simulink model "mcb_param_est_sensorless_nucleo_g474re_ihm07m1"  (R2024a)
settings: Solver=FixedStepDiscrete  StartTime=0.0  StopTime=Inf  FixedStep=Ts  RelTol=1e-3  EnableMultiTasking=on
model workspace (MAT data in the model file):
  encoderResolution = 2000
  hallOffset = '0.5'
  indexOffset = 850
  polePairs = '4'
values from neighbouring files (symbols this model uses):
  PWM_Counter_Period = round(CPU_frequency/PWM_frequency/2)    [mcb_stm32_param_est_InitFunc.m]
  Ts = 1/PWM_frequency    (= 5e-05)    [mcb_stm32_param_est_InitFunc.m]
undefined symbols (not defined in the file or in its folder): DiscIntNeverNeededParam, inverter, motorParam, NumBits1, NumBits2, Slope1, Slope2
libraries: mcbcontrolslib x24, simulink x15, stm32f4xxblockslib x5, stm32g4xxblockslib x4, slpidlib x2, stm32blockslib x2, svdutilitieslib x1
(part 3 of 3)

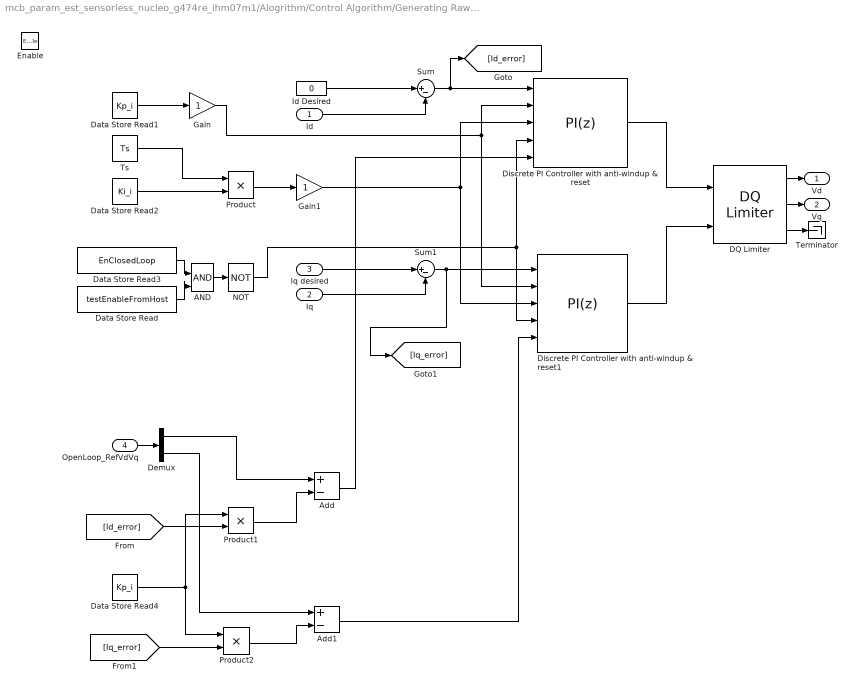
== system mcb_param_est_sensorless_nucleo_g474re_ihm07m1/Alogrithm/Control Algorithm/Generating Raw Space Vectors/OpenLoop_CloseLoop/Control ==
  Id : Inport
  Iq : Inport  Port=2
  Iq desired : Inport  Port=3
  OpenLoop_RefVdVq : Inport  Port=4
  Enable : EnablePort
  AND : Logic  IconShape=distinctive  AllPortsSameDT=off  OutDataTypeStr=boolean
  Add : Sum  Inputs=+-  OutDataTypeStr=single  AccumDataTypeStr=single
  Add1 : Sum  Inputs=+-  OutDataTypeStr=single  AccumDataTypeStr=single
  DQ Limiter : mcbcontrolslib/DQ Limiter  satMethodInputType=Specify via dialog  satMethodSelected=D-Q equivalence  satLimitInputType=Specify via dialog  Vmax=0.95
  Data Store Read : DataStoreRead  DataStoreName=testEnableFromHost  IndexOptions=Index vector (dialog)  Indices=1  OutputSizes=1
  Data Store Read1 : DataStoreRead  DataStoreName=Kp_i  IndexOptions=Index vector (dialog)  Indices=1  OutputSizes=1
  Data Store Read2 : DataStoreRead  DataStoreName=Ki_i  IndexOptions=Index vector (dialog)  Indices=1  OutputSizes=1
  Data Store Read4 : DataStoreRead  DataStoreName=Kp_i  IndexOptions=Index vector (dialog)  Indices=1  OutputSizes=1
  Data Store Read3 : DataStoreRead  DataStoreName=EnClosedLoop  IndexOptions=Index vector (dialog)  Indices=1  OutputSizes=1
  Demux : Demux  Outputs=2
  Discrete PI Controller with anti-windup & reset : slpidlib/PID Controller  Controller=PI  Form=Parallel  TimeDomain=Discrete-time  UseExternalTs=off  SampleTime=-1  IntegratorMethod=Forward Euler  FilterMethod=Forward Euler  ControllerParametersSource=external  P=1  I=1  UseKiTs=on  D=0  UseExternalDerivativeSource=off  N=100  UseFilter=on  TunerSelectOption=Transfer Function Based (PID Tuner App)  InitialConditionSource=external  InitialConditionForIntegrator=0  InitialConditionForFilter=0  DifferentiatorICPrevScaledInput=0  ExternalReset=level  TrackingMode=off  Kt=1  LimitOutput=on  SatLimitsSource=internal  UpperSaturationLimit=1  LowerSaturationLimit=-1  LinearizeAsGain=on  AntiWindupMode=clamping  Kb=1  LimitIntegrator=off  UpperIntegratorSaturationLimit=inf  LowerIntegratorSaturationLimit=-inf  RndMeth=Simplest  POutMin=[]  POutMax=[]  IOutMin=[]  IOutMax=[]  DOutMin=[]  DOutMax=[]  NOutMin=[]  NOutMax=[]  SumOutMin=[]  SumOutMax=[]  SaturationOutDataTypeStr=Inherit: Inherit via back propagation  SaturationOutMin=[]  SaturationOutMax=[]  PParamMin=[]  PParamMax=[]  IParamMin=[]  IParamMax=[]  DParamMin=[]  DParamMax=[]  NParamMin=[]  NParamMax=[]  KbParamMin=[]  KbParamMax=[]  KtParamMin=[]  KtParamMax=[]  KbOutMin=[]  KbOutMax=[]  KtOutMin=[]  KtOutMax=[]  IntegratorOutMin=[]  IntegratorOutMax=[]  FilterOutMin=[]  FilterOutMax=[]  SumI1OutMin=[]  SumI1OutMax=[]  SumI2OutMin=[]  SumI2OutMax=[]  SumI3OutMin=[]  SumI3OutMax=[]  SumI4OutMin=[]  SumI4OutMax=[]  SumDOutMin=[]  SumDOutMax=[]  DifferentiatorOutMin=[]  DifferentiatorOutMax=[]  FilterDiffOutCoefMin=[]  FilterDiffOutCoefMax=[]  ReciprocalOutMin=[]  ReciprocalOutMax=[]  SumDenOutMin=[]  SumDenOutMax=[]  SumNumOutMin=[]  SumNumOutMax=[]  DivideOutMin=[]  DivideOutMax=[]  UdiffTsProdOutMin=[]  UdiffTsProdOutMax=[]  NTsProdOutMin=[]  NTsProdOutMax=[]  UintegralTsProdOutMin=[]  UintegralTsProdOutMax=[]  UngainTsProdOutMin=[]  UngainTsProdOutMax=[]  ClampingZeroOutDataTypeStr=Inherit: Inherit via back propagation  ClampingZeroOutMin=[]  ClampingZeroOutMax=[]  FilterDenConstantOutDataTypeStr=Inherit: Inherit via back propagation  FilterDenConstantOutMin=[]  FilterDenConstantOutMax=[]  PCopyOutDataTypeStr=Inherit: Inherit via back propagation  PCopyOutMin=[]  PCopyOutMax=[]  NCopyOutDataTypeStr=Inherit: Inherit via back propagation  NCopyOutMin=[]  NCopyOutMax=[]  IntegratorContinuousStateAttributes=''  IntegratorStateMustResolveToSignalObject=off  IntegratorRTWStateStorageClass=Auto  FilterContinuousStateAttributes=''  FilterStateMustResolveToSignalObject=off  FilterRTWStateStorageClass=Auto  ParallelPVariant=ExternalParameters  IdealPVariant=Disabled  IVariant=ExternalParameters  DVariant=Disabled  IntegratorVariant=Discrete  SatVariant=Enabled  AWVariant=DiscClampingParallel  PCopyVariant=Disabled  TRVariant=Disabled  FdbkBlocksVariant=Forward  IdealPFdbkVariant=Disabled  SatFdbkVariant=Disabled  DerivativeFilterVariant=Disabled  NVariant=Disabled  NCopyVariant=Disabled_SignalSpec  FilterICVariant=Disabled  IntegratorICVariant=ExternalICs  ExternalResetVariant=ExternalReset  TRSumVariant=Passthrough  SumFdbkVariant=Disabled  SumVariant=Sum_PI  TsampFilterVariant=InternalTs  TsampNgainVariant=Passthrough  TsampIntegralVariant=Disabled_SignalSpec  ExternalSaturationOutDataTypeStr=Inherit: Same as second input  DerivativeSourceVariant=Disabled
  Discrete PI Controller with anti-windup & reset1 : slpidlib/PID Controller  Controller=PI  Form=Parallel  TimeDomain=Discrete-time  UseExternalTs=off  SampleTime=-1  IntegratorMethod=Forward Euler  FilterMethod=Forward Euler  ControllerParametersSource=external  P=1  I=1  UseKiTs=on  D=0  UseExternalDerivativeSource=off  N=100  UseFilter=on  TunerSelectOption=Transfer Function Based (PID Tuner App)  InitialConditionSource=external  InitialConditionForIntegrator=0  InitialConditionForFilter=0  DifferentiatorICPrevScaledInput=0  ExternalReset=level  TrackingMode=off  Kt=1  LimitOutput=on  SatLimitsSource=internal  UpperSaturationLimit=1  LowerSaturationLimit=-1  LinearizeAsGain=on  AntiWindupMode=clamping  Kb=1  LimitIntegrator=off  UpperIntegratorSaturationLimit=inf  LowerIntegratorSaturationLimit=-inf  RndMeth=Simplest  POutMin=[]  POutMax=[]  IOutMin=[]  IOutMax=[]  DOutMin=[]  DOutMax=[]  NOutMin=[]  NOutMax=[]  SumOutMin=[]  SumOutMax=[]  SaturationOutDataTypeStr=Inherit: Inherit via back propagation  SaturationOutMin=[]  SaturationOutMax=[]  PParamMin=[]  PParamMax=[]  IParamMin=[]  IParamMax=[]  DParamMin=[]  DParamMax=[]  NParamMin=[]  NParamMax=[]  KbParamMin=[]  KbParamMax=[]  KtParamMin=[]  KtParamMax=[]  KbOutMin=[]  KbOutMax=[]  KtOutMin=[]  KtOutMax=[]  IntegratorOutMin=[]  IntegratorOutMax=[]  FilterOutMin=[]  FilterOutMax=[]  SumI1OutMin=[]  SumI1OutMax=[]  SumI2OutMin=[]  SumI2OutMax=[]  SumI3OutMin=[]  SumI3OutMax=[]  SumI4OutMin=[]  SumI4OutMax=[]  SumDOutMin=[]  SumDOutMax=[]  DifferentiatorOutMin=[]  DifferentiatorOutMax=[]  FilterDiffOutCoefMin=[]  FilterDiffOutCoefMax=[]  ReciprocalOutMin=[]  ReciprocalOutMax=[]  SumDenOutMin=[]  SumDenOutMax=[]  SumNumOutMin=[]  SumNumOutMax=[]  DivideOutMin=[]  DivideOutMax=[]  UdiffTsProdOutMin=[]  UdiffTsProdOutMax=[]  NTsProdOutMin=[]  NTsProdOutMax=[]  UintegralTsProdOutMin=[]  UintegralTsProdOutMax=[]  UngainTsProdOutMin=[]  UngainTsProdOutMax=[]  ClampingZeroOutDataTypeStr=Inherit: Inherit via back propagation  ClampingZeroOutMin=[]  ClampingZeroOutMax=[]  FilterDenConstantOutDataTypeStr=Inherit: Inherit via back propagation  FilterDenConstantOutMin=[]  FilterDenConstantOutMax=[]  PCopyOutDataTypeStr=Inherit: Inherit via back propagation  PCopyOutMin=[]  PCopyOutMax=[]  NCopyOutDataTypeStr=Inherit: Inherit via back propagation  NCopyOutMin=[]  NCopyOutMax=[]  IntegratorContinuousStateAttributes=''  IntegratorStateMustResolveToSignalObject=off  IntegratorRTWStateStorageClass=Auto  FilterContinuousStateAttributes=''  FilterStateMustResolveToSignalObject=off  FilterRTWStateStorageClass=Auto  ParallelPVariant=ExternalParameters  IdealPVariant=Disabled  IVariant=ExternalParameters  DVariant=Disabled  IntegratorVariant=Discrete  SatVariant=Enabled  AWVariant=DiscClampingParallel  PCopyVariant=Disabled  TRVariant=Disabled  FdbkBlocksVariant=Forward  IdealPFdbkVariant=Disabled  SatFdbkVariant=Disabled  DerivativeFilterVariant=Disabled  NVariant=Disabled  NCopyVariant=Disabled_SignalSpec  FilterICVariant=Disabled  IntegratorICVariant=ExternalICs  ExternalResetVariant=ExternalReset  TRSumVariant=Passthrough  SumFdbkVariant=Disabled  SumVariant=Sum_PI  TsampFilterVariant=InternalTs  TsampNgainVariant=Passthrough  TsampIntegralVariant=Disabled_SignalSpec  ExternalSaturationOutDataTypeStr=Inherit: Same as second input  DerivativeSourceVariant=Disabled
  Gain : Gain  OutDataTypeStr=Inherit: Same as input  ParamDataTypeStr=Inherit: Same as input
  Gain1 : Gain  OutDataTypeStr=Inherit: Same as input  ParamDataTypeStr=Inherit: Same as input
  Id Desired : Constant  Value=0  OutDataTypeStr=single
  NOT : Logic  Operator=NOT  AllPortsSameDT=off  OutDataTypeStr=boolean
  Product : Product  OutDataTypeStr=Inherit: Same as first input
  Product1 : Product  OutDataTypeStr=single
  Product2 : Product  OutDataTypeStr=single
  Sum : Sum  Inputs=|+-
  Sum1 : Sum  Inputs=|+-
  Terminator : Terminator
  Ts : Constant  Value=Ts  OutDataTypeStr=single  SampleTime=-1
  Vd : Outport  VectorParamsAs1DForOutWhenUnconnected=off
  Vq : Outport  Port=2  VectorParamsAs1DForOutWhenUnconnected=off
  wires:
  Id/1 -> Sum/2
  Iq/1 -> Sum1/2
  Iq desired/1 -> Sum1/1
  Id Desired/1 -> Sum/1
  Sum1/1 -> [Iq_error], Discrete PI Controller with anti-windup & reset1/1
  Sum/1 -> [Id_error], Discrete PI Controller with anti-windup & reset/1
  Product/1 -> Gain1/1
  Data Store Read3/1 -> AND/1
  NOT/1 -> Discrete PI Controller with anti-windup & reset/4, Discrete PI Controller with anti-windup & reset1/4
  Data Store Read1/1 -> Gain/1
  Ts/1 -> Product/1
  Data Store Read2/1 -> Product/2
  Discrete PI Controller with anti-windup & reset/1 -> DQ Limiter/1
  Data Store Read/1 -> AND/2
  AND/1 -> NOT/1
  DQ Limiter/1 -> Vd/1
  DQ Limiter/2 -> Vq/1
  DQ Limiter/3 -> Terminator/1
  Discrete PI Controller with anti-windup & reset1/1 -> DQ Limiter/2
  Gain/1 -> Discrete PI Controller with anti-windup & reset/2, Discrete PI Controller with anti-windup & reset1/2
  Gain1/1 -> Discrete PI Controller with anti-windup & reset/3, Discrete PI Controller with anti-windup & reset1/3
  OpenLoop_RefVdVq/1 -> Demux/1
  Demux/2 -> Add1/1
  Demux/1 -> Add/1
  Data Store Read4/1 -> Product1/1, Product2/1
  Product1/1 -> Add/2
  Add/1 -> Discrete PI Controller with anti-windup & reset/5
  Product2/1 -> Add1/2
  Add1/1 -> Discrete PI Controller with anti-windup & reset1/5
  [Id_error] -> Product1/2
  [Iq_error] -> Product2/2

== system mcb_param_est_sensorless_nucleo_g474re_ihm07m1/Alogrithm/Control Algorithm/Generating Raw Space Vectors/OpenLoop_CloseLoop/OpenLoop ==
  TestNum : Inport
  Freq : Inport  Port=2
  RefSignal : Inport  Port=3
  RefSignal_1 : Inport  Port=4
  Enable : EnablePort
  ADC_Calibration : Subsystem
  BiasedSineWaveLdMeas : Subsystem
  Demux : Demux  Outputs=2
  Index Vector : MultiPortSwitch  DataPortOrder=Zero-based contiguous  Inputs=4  zeroidx=on  SaturateOnIntegerOverflow=off  InputSameDT=off
  Rs_Measurement : Subsystem
  SineWaveLqMeas : Subsystem
  RefVd : Outport  VectorParamsAs1DForOutWhenUnconnected=off
  RefVq : Outport  Port=2  VectorParamsAs1DForOutWhenUnconnected=off
  wires:
  Demux/1 -> RefVd/1
  Demux/2 -> RefVq/1
  BiasedSineWaveLdMeas/1(RefVdVq) -> Index Vector/4
  Freq/1 -> SineWaveLqMeas/2(Freq), BiasedSineWaveLdMeas/2(Freq)
  TestNum/1 -> Index Vector/1
  Index Vector/1 -> Demux/1
  Rs_Measurement/1(RefVdVq) -> Index Vector/3  "Rs_Measurement:1"
  ADC_Calibration/1(RefVdVq) -> Index Vector/2  "ADC_Calibration:1"
  RefSignal/1 -> Rs_Measurement/1(Vd_ref), BiasedSineWaveLdMeas/1(Vd_ref), SineWaveLqMeas/1(Vd_ref)
  SineWaveLqMeas/1(RefVdVq) -> Index Vector/5
  RefSignal_1/1 -> SineWaveLqMeas/3(Vdq_amp), BiasedSineWaveLdMeas/3(Vdq_amp)

== system mcb_param_est_sensorless_nucleo_g474re_ihm07m1/Alogrithm/SaveEstParam_Serial Send/Serial Send/AlternateData/Alternate_0_2 ==
  NOT : Logic  Operator=NOT  IconShape=distinctive  AllPortsSameDT=off  OutDataTypeStr=boolean
  Unit Delay : UnitDelay  InitialCondition=1  SampleTime=-1  HasFrameUpgradeWarning=on
  Out1 : Outport
  wires:
  NOT/1 -> Unit Delay/1, Out1/1
  Unit Delay/1 -> NOT/1

== system mcb_param_est_sensorless_nucleo_g474re_ihm07m1/Alogrithm/SaveEstParam_Serial Send/Serial Send/Serial Send/Data ==
  Data : Inport
  Data_width : Inport  Port=2
  Action Port : ActionPort  ActionPortLabel=else
  Mux : Mux  Inputs=2
  Start : Constant  Value=hex2dec('00000000')  OutDataTypeStr=uint32
  Data_out : Outport  VectorParamsAs1DForOutWhenUnconnected=off
  Iteration : Outport  Port=2  VectorParamsAs1DForOutWhenUnconnected=off
  wires:
  Start/1 -> Mux/2
  Mux/1 -> Data_out/1
  Data/1 -> Mux/1
  Data_width/1 -> Iteration/1

== system mcb_param_est_sensorless_nucleo_g474re_ihm07m1/Alogrithm/SaveEstParam_Serial Send/Serial Send/Serial Send/End ==
  Data : Inport
  Data_width : Inport  Port=2
  Action Port : ActionPort  ActionPortLabel=elseif(u1 == 599)
  Bias : Bias  Bias=1  SaturateOnIntegerOverflow=off
  Mux : Mux  Inputs=2
  Start : Constant  Value=hex2dec('45454545')  OutDataTypeStr=uint32
  Data_out : Outport  VectorParamsAs1DForOutWhenUnconnected=off
  Iteration : Outport  Port=2  VectorParamsAs1DForOutWhenUnconnected=off
  wires:
  Mux/1 -> Data_out/1
  Data_width/1 -> Bias/1
  Start/1 -> Mux/2
  Bias/1 -> Iteration/1
  Data/1 -> Mux/1

== system mcb_param_est_sensorless_nucleo_g474re_ihm07m1/Alogrithm/SaveEstParam_Serial Send/Serial Send/Serial Send/Start ==
  Data : Inport
  Data_width : Inport  Port=2
  Action Port : ActionPort  ActionPortLabel=if(u1 == 0)
  Bias : Bias  Bias=1  SaturateOnIntegerOverflow=off
  End : Constant  Value=hex2dec('53535353')  OutDataTypeStr=uint32
  Mux : Mux  Inputs=2
  Data_out : Outport  VectorParamsAs1DForOutWhenUnconnected=off
  Iteration : Outport  Port=2  VectorParamsAs1DForOutWhenUnconnected=off
  wires:
  End/1 -> Mux/1
  Mux/1 -> Data_out/1
  Data_width/1 -> Bias/1
  Bias/1 -> Iteration/1
  Data/1 -> Mux/2

== system mcb_param_est_sensorless_nucleo_g474re_ihm07m1/Alogrithm/SaveEstParam_Serial Send/Serial Send/Serial Send/While Iterator Subsystem ==
  Data : Inport
  Iteration : Inport  Port=2
  Add : Sum  Inputs=+-  OutDataTypeStr=Inherit: Same as first input
  Index Vector : MultiPortSwitch  Inputs=1  SaturateOnIntegerOverflow=off  InputSameDT=off
  UART/USART Write : stm32blockslib/UART//USART Write  Priority=1  UARTModule=LPUART1  LengthOfDataToSend=off  BlockingMode=on  BlockingTimeout=1e-3  OutputStatus=off
  While Iterator : WhileIterator  MaxIters=-1  WhileBlockType=do-while  ShowIterationPort=on  OutputDataType=int16
  wires:
  Iteration/1 -> Add/1
  Add/1 -> While Iterator/1
  Index Vector/1 -> UART/USART Write/1
  Data/1 -> Index Vector/2
  While Iterator/1 -> Index Vector/1, Add/2

== system mcb_param_est_sensorless_nucleo_g474re_ihm07m1/Alogrithm/Control Algorithm/Flux Observer/FluxObvserver/FluxObserverSubsystem/psiAlpha ==
  note: Integrator
  Reset : Inport
  Valpha : Inport  Port=2
  Ialpha : Inport  Port=3
  scaling : Inport  Port=4
  scalingLd : Inport  Port=5
  Data Type Propagation : simulink/Signal Attributes/Data Type Propagation  PropDataType=fixdt(1, 16)  IfRefDouble=double  IfRefSingle=single  IsSigned=IsSigned1 or IsSigned2  NumBitsBase=max([NumBits1 NumBits2])  NumBitsMult=1  NumBitsAdd=0  NumBitsAllowFinal=1:128  PropScalingMode=Obtain via best precision  PropScaling=2^-10  ValuesUsedBestPrec=[4 -4]  SlopeBase=min([Slope1 Slope2])  SlopeMult=1  SlopeAdd=0  BiasBase=Bias1  BiasMult=1  BiasAdd=0
  Delay : Delay  DelayLength=1  ExternalReset=Level
      settings: InputPortMap=u0,r5
  Gain : Gain  Gain=Ts  ParamDataTypeStr=Inherit: Inherit from 'Gain'  OutDataTypeStr=Inherit: Inherit via back propagation
  IIR Filter3 : mcbcontrolslib/IIR Filter  VariantControl=Low Pass Filter  VariantSelect=Low-pass  FilterConstantInputType=Specify via dialog  Filter_constant=0.001*(Ts/(50e-6))  advancedSettings=off  Ts=50e-6  cutOff_freq=1
  Product : Product  RndMeth=Simplest  OutDataTypeStr=Inherit: Same as first input
  Scaling : Subsystem
  Sum : Sum  Inputs=|++
  Sum1 : Sum  Inputs=|+-  RndMeth=Simplest  OutDataTypeStr=Inherit: Same as first input
  Sum3 : Sum  Inputs=|+-  RndMeth=Simplest  OutDataTypeStr=Inherit: Same as first input
  Sum6 : Sum  Inputs=|+-  RndMeth=Simplest  OutDataTypeStr=Inherit: Same as first input
  psiAlpha : Outport
  wires:
  Sum/1 -> Sum1/1, Delay/1
  IIR Filter3/1 -> Sum6/2
  Sum6/1 -> psiAlpha/1
  Valpha/1 -> Scaling/1("Valpha ")
  Ialpha/1 -> Product/1, Scaling/2(Ialpha)
  Scaling/1(ValphaScaled) -> Sum3/1
  Scaling/2(IalphaScaled*R) -> Sum3/2
  Delay/1 -> Sum/2
  Reset/1 -> Delay/2
  Sum3/1 -> Data Type Propagation/2, Data Type Propagation/1, Gain/1
  Gain/1 -> Data Type Propagation/3, Sum/1
  scaling/1 -> Scaling/3(scaling)
  Sum1/1 -> IIR Filter3/1, Sum6/1
  Product/1 -> Sum1/2
  scalingLd/1 -> Product/2

== system mcb_param_est_sensorless_nucleo_g474re_ihm07m1/Alogrithm/Control Algorithm/Flux Observer/FluxObvserver/FluxObserverSubsystem/psiBeta ==
  note: Integrator
  Vbeta : Inport
  Ibeta : Inport  Port=2
  Reset : Inport  Port=3
  scaling : Inport  Port=4
  scalingLd : Inport  Port=5
  Data Type Propagation : simulink/Signal Attributes/Data Type Propagation  PropDataType=fixdt(1, 16)  IfRefDouble=double  IfRefSingle=single  IsSigned=IsSigned1 or IsSigned2  NumBitsBase=max([NumBits1 NumBits2])  NumBitsMult=1  NumBitsAdd=0  NumBitsAllowFinal=1:128  PropScalingMode=Obtain via best precision  PropScaling=2^-10  ValuesUsedBestPrec=[4 -4]  SlopeBase=min([Slope1 Slope2])  SlopeMult=1  SlopeAdd=0  BiasBase=Bias1  BiasMult=1  BiasAdd=0
  Delay : Delay  DelayLength=1  InitialCondition=0  ExternalReset=Level
      settings: InputPortMap=u0,r5
  Gain : Gain  Gain=Ts  ParamDataTypeStr=Inherit: Inherit from 'Gain'  OutDataTypeStr=Inherit: Inherit via back propagation
  IIR Filter : mcbcontrolslib/IIR Filter  VariantControl=Low Pass Filter  VariantSelect=Low-pass  FilterConstantInputType=Specify via dialog  Filter_constant=0.001*(Ts/(50e-6))  advancedSettings=off  Ts=50e-6  cutOff_freq=1
  Product : Product  RndMeth=Simplest  OutDataTypeStr=Inherit: Same as first input
  Scaling : Subsystem
  Sum : Sum  Inputs=|++  OutDataTypeStr=Inherit: Same as first input
  Sum1 : Sum  Inputs=|+-  RndMeth=Simplest  OutDataTypeStr=Inherit: Same as first input
  Sum3 : Sum  Inputs=|+-  RndMeth=Simplest  OutDataTypeStr=Inherit: Same as first input
  Sum6 : Sum  Inputs=|+-  RndMeth=Simplest  OutDataTypeStr=Inherit: Same as first input
  psiBeta : Outport
  wires:
  Sum/1 -> Sum1/1, Delay/1
  IIR Filter/1 -> Sum6/2
  Sum6/1 -> psiBeta/1
  Vbeta/1 -> Scaling/1(Vbeta)
  Ibeta/1 -> Product/1, Scaling/2(Ibeta)
  Scaling/2(IbetaScaled*R) -> Sum3/2
  Scaling/1(VbetaScaled) -> Sum3/1
  Delay/1 -> Sum/2
  Sum3/1 -> Data Type Propagation/2, Data Type Propagation/1, Gain/1
  Gain/1 -> Data Type Propagation/3, Sum/1
  Reset/1 -> Delay/2
  scaling/1 -> Scaling/3(scaling)
  Sum1/1 -> IIR Filter/1, Sum6/1
  Product/1 -> Sum1/2
  scalingLd/1 -> Product/2

== system mcb_param_est_sensorless_nucleo_g474re_ihm07m1/Alogrithm/Control Algorithm/Flux Observer/FluxObvserver/SpeedMeasurementSubsystem/Speed_measurement ==
  note: 60/(DelayLength*SampleTimeAsync(1)*PU_System.N_base*(2^32))
  note: Speed measurement
  PositionPU : Inport
  MaxSpeed : Inport  Port=2
  2^32/2 : Constant  Value=2^31  OutDataTypeStr=single  SampleTime=-1
  Constant : Constant  Value=30  OutDataTypeStr=single
  Delay : Delay  DelayLengthSource=Input port  DelayLength=10  DelayLengthUpperLimit=800  UseCircularBuffer=on
      settings: InputPortMap=u0,p1
  DelayLength : Constant  Value=10  OutDataTypeStr=single  SampleTime=-1
  Divide : Product  Inputs=*/  RndMeth=Simplest  OutDataTypeStr=Inherit: Same as first input
  Product : Product  Inputs=4
  Product1 : Product  OutDataTypeStr=single  RndMeth=Simplest
  SampleTime : Constant  Value=Ts  OutDataTypeStr=single
  SpeedCount : Sum  Inputs=+-|  OutDataTypeStr=int32  RndMeth=Simplest
  SpeedToCount : Gain  Gain=uint32(2^32/1)  ParamDataTypeStr=single  OutDataTypeStr=uint32  RndMeth=Simplest
  speedPU : Outport
  wires:
  SpeedCount/1 -> Product1/1
  SampleTime/1 -> Product/1
  MaxSpeed/1 -> Product/2
  Constant/1 -> Divide/1
  Product/1 -> Divide/2
  SpeedToCount/1 -> SpeedCount/1, Delay/1
  PositionPU/1 -> SpeedToCount/1
  Product1/1 -> speedPU/1
  Delay/1 -> SpeedCount/2
  2^32/2/1 -> Product/3
  DelayLength/1 -> Delay/2, Product/4
  Divide/1 -> Product1/2

== system mcb_param_est_sensorless_nucleo_g474re_ihm07m1/Alogrithm/Control Algorithm/Generating Raw Space Vectors/Open Loop Start-Up/Open Loop Start-Up/Ramp Generator ==
  Ramp_Time : Inport
  Enable : Inport  Port=2
  Divide : Product  Inputs=*/  RndMeth=Simplest  OutDataTypeStr=Inherit: Same as first input
  NOT : Logic  Operator=NOT  IconShape=distinctive  AllPortsSameDT=off  OutDataTypeStr=boolean
  One : Constant  OutDataTypeStr=single  SampleTime=-1
  Ramp Generator : DiscreteIntegrator  IntegratorMethod=Accumulation: Forward Euler  gainval=1  ExternalReset=sampled level  SampleTime=-1  OutDataTypeStr=single  RndMeth=Simplest  LimitOutput=on  UpperSaturationLimit=1  LowerSaturationLimit=0  ICPrevOutput=DiscIntNeverNeededParam  ICPrevScaledInput=DiscIntNeverNeededParam
  Sample_Time : Gain  Gain=Ts  RndMeth=Simplest  OutDataTypeStr=Inherit: Same as input
  Ramp : Outport
  wires:
  Divide/1 -> Sample_Time/1
  Ramp Generator/1 -> Ramp/1  "Eps"
  Sample_Time/1 -> Ramp Generator/1
  One/1 -> Divide/1
  Ramp_Time/1 -> Divide/2
  Enable/1 -> NOT/1
  NOT/1 -> Ramp Generator/2

== system mcb_param_est_sensorless_nucleo_g474re_ihm07m1/Alogrithm/Control Algorithm/Generating Raw Space Vectors/Open Loop Start-Up/Open Loop Start-Up/V-by-f ==
  Frequency : Inport
  Data Store Read3 : DataStoreRead  DataStoreName=pole_pairs  IndexOptions=Index vector (dialog)  Indices=1  OutputSizes=1
  Data Store Read4 : DataStoreRead  DataStoreName=speed_rated  IndexOptions=Index vector (dialog)  Indices=1  OutputSizes=1
  Divide : Product  Inputs=*/  OutDataTypeStr=Inherit: Same as first input
  Product2 : Product
  V-by-f : Gain  Gain=60  RndMeth=Simplest  OutDataTypeStr=Inherit: Same as input
  speedPU : Outport
  wires:
  Divide/1 -> speedPU/1
  Frequency/1 -> V-by-f/1
  V-by-f/1 -> Divide/1
  Product2/1 -> Divide/2
  Data Store Read4/1 -> Product2/2
  Data Store Read3/1 -> Product2/1

== system mcb_param_est_sensorless_nucleo_g474re_ihm07m1/Alogrithm/Control Algorithm/Generating Raw Space Vectors/OpenLoop_CloseLoop/OpenLoop/ADC_Calibration ==
  Constant1 : Constant  Value=0  OutDataTypeStr=single  SampleTime=-1
  Constant2 : Constant  Value=0  OutDataTypeStr=single  SampleTime=-1
  Mux : Mux  Inputs=2
  RefVdVq : Outport  VectorParamsAs1DForOutWhenUnconnected=off
  wires:
  Constant2/1 -> Mux/2
  Constant1/1 -> Mux/1
  Mux/1 -> RefVdVq/1

== system mcb_param_est_sensorless_nucleo_g474re_ihm07m1/Alogrithm/Control Algorithm/Generating Raw Space Vectors/OpenLoop_CloseLoop/OpenLoop/BiasedSineWaveLdMeas ==
  Vd_ref : Inport
  Freq : Inport  Port=2
  Vdq_amp : Inport  Port=3
  Constant1 : Constant  Value=0  OutDataTypeStr=single  SampleTime=-1
  Mux : Mux  Inputs=2
  Sine2 : Subsystem
  RefVdVq : Outport  VectorParamsAs1DForOutWhenUnconnected=off
  wires:
  Constant1/1 -> Mux/2
  Mux/1 -> RefVdVq/1
  Freq/1 -> Sine2/1(Freq)
  Vd_ref/1 -> Sine2/2(Vd_dc)
  Sine2/1(sinBiased) -> Mux/1
  Vdq_amp/1 -> Sine2/3(Vdq_amp)

== system mcb_param_est_sensorless_nucleo_g474re_ihm07m1/Alogrithm/Control Algorithm/Generating Raw Space Vectors/OpenLoop_CloseLoop/OpenLoop/Rs_Measurement ==
  Vd_ref : Inport
  Mux1 : Mux  Inputs=2
  Vq_ref : Constant  Value=0  OutDataTypeStr=single  SampleTime=-1
  RefVdVq : Outport  VectorParamsAs1DForOutWhenUnconnected=off
  wires:
  Vq_ref/1 -> Mux1/2
  Vd_ref/1 -> Mux1/1
  Mux1/1 -> RefVdVq/1

== system mcb_param_est_sensorless_nucleo_g474re_ihm07m1/Alogrithm/Control Algorithm/Generating Raw Space Vectors/OpenLoop_CloseLoop/OpenLoop/SineWaveLqMeas ==
  Vd_ref : Inport
  Freq : Inport  Port=2
  Vdq_amp : Inport  Port=3
  Mux : Mux  Inputs=2
  Sine3 : Subsystem
  RefVdVq : Outport  VectorParamsAs1DForOutWhenUnconnected=off
  wires:
  Mux/1 -> RefVdVq/1
  Vd_ref/1 -> Mux/1
  Freq/1 -> Sine3/1(Freq)
  Sine3/1(sin) -> Mux/2
  Vdq_amp/1 -> Sine3/2(Vdq_amp)

== system mcb_param_est_sensorless_nucleo_g474re_ihm07m1/Alogrithm/Control Algorithm/Flux Observer/FluxObvserver/FluxObserverSubsystem/psiAlpha/Scaling ==
  "Valpha " : Inport
  Ialpha : Inport  Port=2
  scaling : Inport  Port=3
  Product : Product  RndMeth=Simplest  OutDataTypeStr=Inherit: Same as first input
  ValphaScaled : Outport
  IalphaScaled*R : Outport  Port=2
  wires:
  Ialpha/1 -> Product/1
  Product/1 -> IalphaScaled*R/1
  "Valpha "/1 -> ValphaScaled/1
  scaling/1 -> Product/2

== system mcb_param_est_sensorless_nucleo_g474re_ihm07m1/Alogrithm/Control Algorithm/Flux Observer/FluxObvserver/FluxObserverSubsystem/psiBeta/Scaling ==
  Vbeta : Inport
  Ibeta : Inport  Port=2
  scaling : Inport  Port=3
  Product : Product  RndMeth=Simplest  OutDataTypeStr=Inherit: Same as first input
  VbetaScaled : Outport
  IbetaScaled*R : Outport  Port=2
  wires:
  Product/1 -> IbetaScaled*R/1
  Vbeta/1 -> VbetaScaled/1
  scaling/1 -> Product/2
  Ibeta/1 -> Product/1

== system mcb_param_est_sensorless_nucleo_g474re_ihm07m1/Alogrithm/Control Algorithm/Generating Raw Space Vectors/OpenLoop_CloseLoop/OpenLoop/BiasedSineWaveLdMeas/Sine2 ==
  note: Vdq_amp * sin(2 * pi * Freq * n * Ts))+Sine_Vdc
  Freq : Inport
  Vd_dc : Inport  Port=2
  Vdq_amp : Inport  Port=3
  Gain : Gain  Gain=Ts
  Position Generator : mcbcontrolslib/Position Generator  AngleOutput=Per-unit  ExternalReset=none  Offset=0
  Product : Product
  Sine-Cosine Lookup : mcbcontrolslib/Sine-Cosine Lookup  AngleInput=Per-unit  N_points=1024  DatatypeInput=Inherit from input  Datatype=single
  Sum : Sum  Inputs=|++
  Terminator : Terminator
  sinBiased : Outport  VectorParamsAs1DForOutWhenUnconnected=off
  wires:
  Product/1 -> Sum/1
  Sine-Cosine Lookup/2 -> Terminator/1
  Sine-Cosine Lookup/1 -> Product/1
  Sum/1 -> sinBiased/1
  Freq/1 -> Gain/1
  Gain/1 -> Position Generator/1
  Vdq_amp/1 -> Product/2
  Vd_dc/1 -> Sum/2
  Position Generator/1 -> Sine-Cosine Lookup/1  "Eps"

== system mcb_param_est_sensorless_nucleo_g474re_ihm07m1/Alogrithm/Control Algorithm/Generating Raw Space Vectors/OpenLoop_CloseLoop/OpenLoop/SineWaveLqMeas/Sine3 ==
  note: Vdq_amp * sin(2 * pi * Freq * n * Ts))
  Freq : Inport
  Vdq_amp : Inport  Port=2
  Gain : Gain  Gain=Ts
  Position Generator : mcbcontrolslib/Position Generator  AngleOutput=Per-unit  ExternalReset=none  Offset=0
  Product : Product
  Sine-Cosine Lookup : mcbcontrolslib/Sine-Cosine Lookup  AngleInput=Per-unit  N_points=1024  DatatypeInput=Inherit from input  Datatype=single
  Terminator : Terminator
  sin : Outport  VectorParamsAs1DForOutWhenUnconnected=off
  wires:
  Sine-Cosine Lookup/2 -> Terminator/1
  Sine-Cosine Lookup/1 -> Product/1
  Product/1 -> sin/1
  Freq/1 -> Gain/1
  Gain/1 -> Position Generator/1
  Vdq_amp/1 -> Product/2
  Position Generator/1 -> Sine-Cosine Lookup/1  "Eps"

== matlab function mcb_param_est_sensorless_nucleo_g474re_ihm07m1/Alogrithm/ParameterEstimationTests/MATLAB Function ==
  data: AlgoParams input; SignalsPU input size=6; Ts input; curTime input single; RsMeasTestTime input; testNumOut output; injFreqOut output; refSignalOut output; refSignalOut1 output; estimatedParameterOut output; I_rated input; pole_pairs input; Rs input; Ld input; R_board input; testEnableOut output; V_rated input; estParIdxOut output; currentPU_RWV input; sigma input; Kp_iOut output; Ki_iOut output; IaIbVdc input; inverter_V_max input; speedFB input; speed_rated input; PhaseDiff output
function [testNumOut, injFreqOut, refSignalOut, refSignalOut1, estimatedParameterOut, testEnableOut, estParIdxOut, Kp_iOut, Ki_iOut, PhaseDiff] = fcn(AlgoParams, SignalsPU, Ts, curTime, RsMeasTestTime, I_rated, pole_pairs, Rs, Ld, R_board, V_rated, currentPU_RWV, sigma, IaIbVdc, inverter_V_max, speedFB, speed_rated)
coder.allowpcode('plain'); 
%#codegen
[testNumOut, injFreqOut, refSignalOut, refSignalOut1, estimatedParameterOut, testEnableOut, estParIdxOut, Kp_iOut, Ki_iOut, PhaseDiff] = mcb.internal.estimateMotorParam(AlgoParams, SignalsPU, Ts, curTime, RsMeasTestTime, I_rated, pole_pairs, Rs, Ld, R_board, V_rated, currentPU_RWV, sigma, IaIbVdc, inverter_V_max, speedFB, speed_rated);
